simulink model "isprobavenje_persistent"  (R2018b)
settings: Solver=VariableStepAuto  StartTime=0.0  StopTime=10.0  RelTol=1e-3
settings Model: Creator=branko  LastModifiedBy=branko

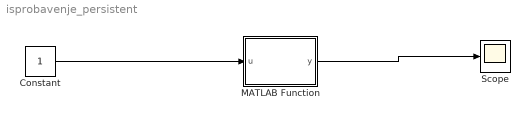
== system isprobavenje_persistent ==
  Constant : Constant  OutDataTypeStr=int16  SampleTime=-1
  MATLAB Function : MATLAB Function  TreatAsAtomicUnit=on  SystemSampleTime=0.01
  Scope : Scope
  wires:
  Constant/1 -> MATLAB Function/1(u)
  MATLAB Function/1(y) -> Scope/1

== matlab function isprobavenje_persistent/MATLAB Function ==
  data: u input; y output
function y = fcn(u)

persistent a
if isempty (a)
   a=1.0;
end
a = a+1.0;
y = u*a;
end
